simulink model "pitchPIDsimulation"  (R2025b)
settings: Solver=VariableStepAuto  StartTime=0.0  StopTime=15  RelTol=1e-3
undefined symbols (not defined in the file): CG, LongInertia, Mass, RotateInertia, Time
libraries: simulink x2, slpidlib x1
settings Model: Creator=Alienware R7  LastModifiedBy=Alienware R7

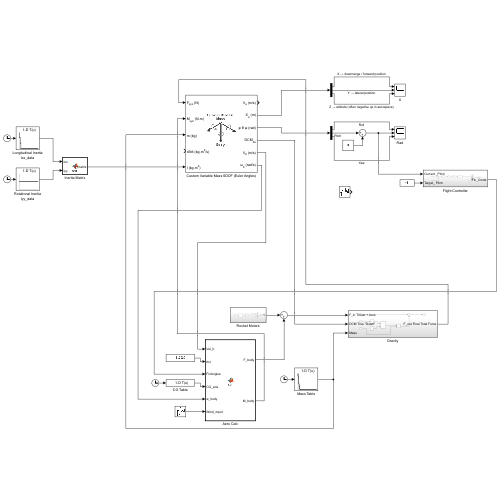
[thumbnail: Simulink's stored preview of the top-level diagram]
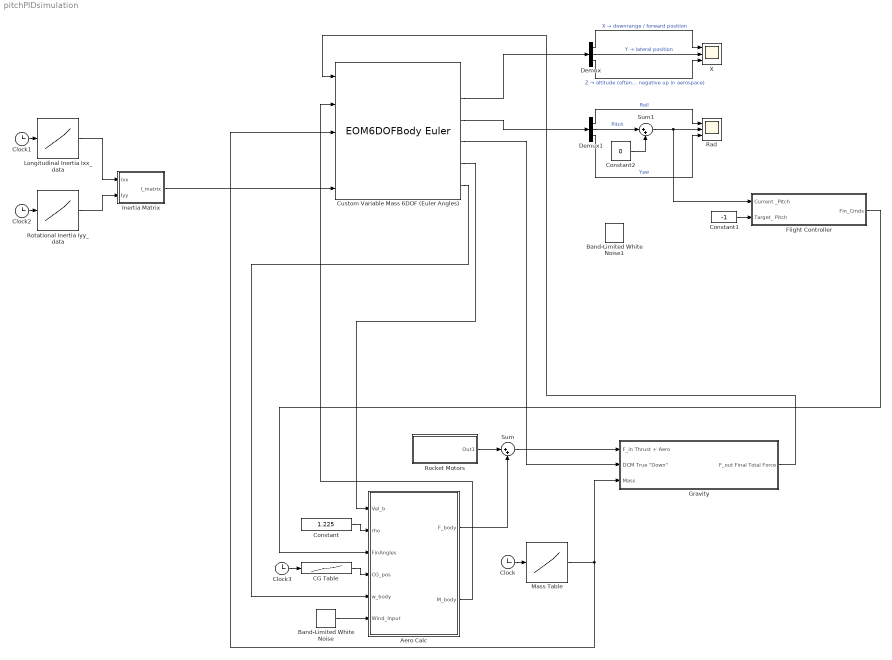
== system pitchPIDsimulation ==
  Aero Calc : MATLAB Function  TreatAsAtomicUnit=on
  Band-Limited White Noise : simulink/Sources/Band-Limited White Noise  Cov=0.1  Ts=0.05  seed=[23341]
  Band-Limited White Noise1 : simulink/Sources/Band-Limited White Noise  Cov=0.00005  Ts=0.01  seed=[23341]
  CG Table : Lookup_n-D  NumberOfTableDimensions=1  BreakpointsForDimension1=Time  Table=CG  InternalRulePriority=Speed  RndMeth=Simplest
  Clock{,1..3} (4 alike) : Clock
  Constant : Constant  Value=1.225
  Constant1 : Constant  Value=-1
  Constant2 : Constant  Value=0
  Custom Variable Mass 6DOF (Euler Angles) : EOM6DOFBodyEuler  mtype=Custom Variable  eul_0=[0 -0.75 0]
  Demux : Demux  Outputs=3
  Demux1 : Demux  Outputs=3
  Flight Controller : Subsystem
  Gravity : Subsystem
  Inertia Matrix : MATLAB Function  TreatAsAtomicUnit=on
  Longitudinal Inertia Ixx_data : Lookup_n-D  NumberOfTableDimensions=1  BreakpointsForDimension1=Time  Table=LongInertia  InternalRulePriority=Speed  RndMeth=Simplest
  Mass Table : Lookup_n-D  NumberOfTableDimensions=1  BreakpointsForDimension1=Time  Table=Mass  InternalRulePriority=Speed  RndMeth=Simplest
  Rad : Scope  NumInputPorts=3
      settings: ActiveDisplayYMinimum=-4.2416234281140159  ActiveDisplayYMaximum=2.850977580357458
  Rocket Motors : Subsystem
  Rotational Inertia Iyy_data : Lookup_n-D  NumberOfTableDimensions=1  BreakpointsForDimension1=Time  Table=RotateInertia  InternalRulePriority=Speed  RndMeth=Simplest
  Sum : Sum  Inputs=|++
  Sum1 : Sum  Inputs=|++
  X : Scope  NumInputPorts=3
      settings: ActiveDisplayYMinimum=-21.697738023426126  ActiveDisplayYMaximum=401.42440236350615
  wires:
  Rocket Motors/1(Out1) -> Sum/1
  Longitudinal Inertia Ixx_data/1 -> Inertia Matrix/1(Ixx)
  Rotational Inertia Iyy_data/1 -> Inertia Matrix/2(Iyy)
  Custom Variable Mass 6DOF (Euler Angles)/5 -> Aero Calc/1(Vel_b)
  CG Table/1 -> Aero Calc/4(CG_pos)
  Constant/1 -> Aero Calc/2(rho)
  Aero Calc/1(F_body) -> Sum/2
  Sum/1 -> Gravity/1(F_in Thrust + Aero)
  Custom Variable Mass 6DOF (Euler Angles)/4 -> Gravity/2("DCM True \"Down\"")
  Mass Table/1 -> Custom Variable Mass 6DOF (Euler Angles)/3, Gravity/3(Mass)
  Gravity/1(F_out Final Total Force) -> Custom Variable Mass 6DOF (Euler Angles)/1
  Clock/1 -> Mass Table/1
  Clock1/1 -> Longitudinal Inertia Ixx_data/1
  Clock2/1 -> Rotational Inertia Iyy_data/1
  Clock3/1 -> CG Table/1
  Inertia Matrix/1(I_matrix) -> Custom Variable Mass 6DOF (Euler Angles)/5
  Demux1/1 -> Rad/1  "Roll"
  Demux/2 -> X/2  "Y → lateral position"
  Demux1/3 -> Rad/3  "Yaw"
  Demux/3 -> X/3  "Z → altitude (often negative up in aerospace)"
  Demux/1 -> X/1  "X → downrange / forward position"
  Flight Controller/1(Fin_Cmds) -> Aero Calc/3(FinAngles)
  Aero Calc/2(M_body) -> Custom Variable Mass 6DOF (Euler Angles)/2
  Custom Variable Mass 6DOF (Euler Angles)/6 -> Aero Calc/5(w_body)
  Custom Variable Mass 6DOF (Euler Angles)/2 -> Demux/1
  Custom Variable Mass 6DOF (Euler Angles)/3 -> Demux1/1
  Demux1/2 -> Sum1/1  "Pitch"
  Sum1/1 -> Flight Controller/1(Current _Pitch), Rad/2
  Band-Limited White Noise/1 -> Aero Calc/6(Wind_Input)
  Constant1/1 -> Flight Controller/2(Target_ Pitch)
  Constant2/1 -> Sum1/2

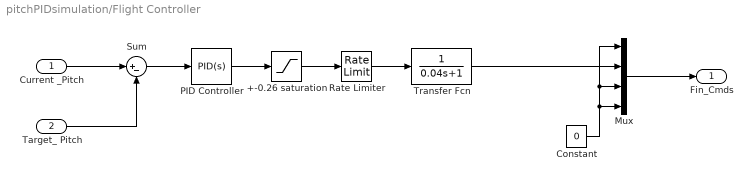
== system pitchPIDsimulation/Flight Controller ==
  Current _Pitch : Inport
  Target_ Pitch : Inport  Port=2
  +-0.26 saturation : Saturate  UpperLimit=0.26  LowerLimit=-0.26
  Constant : Constant  Value=0
  Mux : Mux
  PID Controller : slpidlib/PID Controller  Controller=PID  Form=Parallel  TimeDomain=Continuous-time  UseExternalTs=off  SampleTime=-1  IntegratorMethod=Forward Euler  FilterMethod=Forward Euler  ControllerParametersSource=internal  P=0.4  I=0  UseKiTs=off  D=0  UseExternalDerivativeSource=off  N=100  UseFilter=on  TunerSelectOption=Transfer Function Based (PID Tuner App)  InitialConditionSource=internal  InitialConditionForIntegrator=0  InitialConditionForFilter=0  DifferentiatorICPrevScaledInput=0  ExternalReset=none  TrackingMode=off  Kt=1  LimitOutput=off  SatLimitsSource=internal  UpperSaturationLimit=inf  LowerSaturationLimit=-inf  LinearizeAsGain=on  AntiWindupMode=none  Kb=1  LimitIntegrator=off  UpperIntegratorSaturationLimit=inf  LowerIntegratorSaturationLimit=-inf  POutMin=[]  POutMax=[]  IOutMin=[]  IOutMax=[]  DOutMin=[]  DOutMax=[]  NOutMin=[]  NOutMax=[]  SumOutMin=[]  SumOutMax=[]  SaturationOutMin=[]  SaturationOutMax=[]  PParamMin=[]  PParamMax=[]  IParamMin=[]  IParamMax=[]  DParamMin=[]  DParamMax=[]  NParamMin=[]  NParamMax=[]  KbParamMin=[]  KbParamMax=[]  KtParamMin=[]  KtParamMax=[]  KbOutMin=[]  KbOutMax=[]  KtOutMin=[]  KtOutMax=[]  IntegratorOutMin=[]  IntegratorOutMax=[]  FilterOutMin=[]  FilterOutMax=[]  SumI1OutMin=[]  SumI1OutMax=[]  SumI2OutMin=[]  SumI2OutMax=[]  SumI3OutMin=[]  SumI3OutMax=[]  SumI4OutMin=[]  SumI4OutMax=[]  SumDOutMin=[]  SumDOutMax=[]  DifferentiatorOutMin=[]  DifferentiatorOutMax=[]  FilterDiffOutCoefMin=[]  FilterDiffOutCoefMax=[]  ReciprocalOutMin=[]  ReciprocalOutMax=[]  SumDenOutMin=[]  SumDenOutMax=[]  SumNumOutMin=[]  SumNumOutMax=[]  DivideOutMin=[]  DivideOutMax=[]  UdiffTsProdOutMin=[]  UdiffTsProdOutMax=[]  NTsProdOutMin=[]  NTsProdOutMax=[]  UintegralTsProdOutMin=[]  UintegralTsProdOutMax=[]  UngainTsProdOutMin=[]  UngainTsProdOutMax=[]  ClampingZeroOutDataTypeStr=Inherit: Inherit via back propagation  ClampingZeroOutMin=[]  ClampingZeroOutMax=[]  FilterDenConstantOutDataTypeStr=Inherit: Inherit via back propagation  FilterDenConstantOutMin=[]  FilterDenConstantOutMax=[]  PCopyOutDataTypeStr=Inherit: Inherit via back propagation  PCopyOutMin=[]  PCopyOutMax=[]  NCopyOutDataTypeStr=Inherit: Inherit via back propagation  NCopyOutMin=[]  NCopyOutMax=[]  IntegratorContinuousStateAttributes=''  IntegratorStateMustResolveToSignalObject=off  IntegratorRTWStateStorageClass=Auto  FilterContinuousStateAttributes=''  FilterStateMustResolveToSignalObject=off  FilterRTWStateStorageClass=Auto  ParallelPVariant=InternalParameters  IdealPVariant=Disabled  IVariant=InternalParameters  DVariant=InternalParameters  IntegratorVariant=Continuous  SatVariant=Disabled  AWVariant=Passthrough  PCopyVariant=Disabled  TRVariant=Disabled  FdbkBlocksVariant=Forward  IdealPFdbkVariant=Disabled  SatFdbkVariant=Disabled  DerivativeFilterVariant=ContFilter  NVariant=InternalParameters  NCopyVariant=Disabled  FilterICVariant=InternalICsFilter  IntegratorICVariant=InternalICs  ExternalResetVariant=Disabled  TRSumVariant=Passthrough  SumFdbkVariant=Disabled  SumVariant=Sum_PID  TsampFilterVariant=InternalTs  TsampNgainVariant=Passthrough  TsampIntegralVariant=Disabled_SignalSpec  ExternalSaturationOutDataTypeStr=Inherit: Same as second input  DerivativeSourceVariant=ErrorSignal  PreIntVariant=InternalPreInt
  Rate Limiter : RateLimiter  RisingSlewLimit=8.05  FallingSlewLimit=-8.05  SampleTimeMode=inherited
  Sum : Sum  Inputs=|+-
  Transfer Fcn : TransferFcn  Denominator=[0.04 1]
  Fin_Cmds : Outport
  wires:
  Target_ Pitch/1 -> Sum/2
  Current _Pitch/1 -> Sum/1
  Sum/1 -> PID Controller/1
  PID Controller/1 -> +-0.26 saturation/1
  +-0.26 saturation/1 -> Rate Limiter/1
  Constant/1 -> Mux/3, Mux/1, Mux/4
  Mux/1 -> Fin_Cmds/1
  Rate Limiter/1 -> Transfer Fcn/1
  Transfer Fcn/1 -> Mux/2

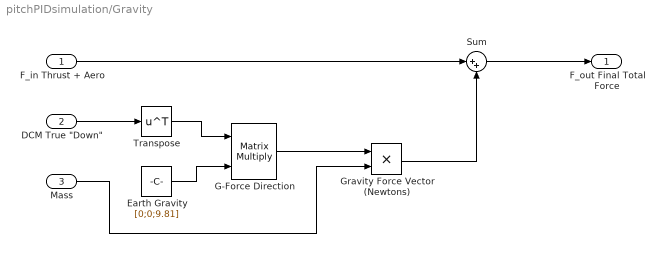
== system pitchPIDsimulation/Gravity ==
  F_in Thrust + Aero : Inport
  "DCM True \"Down\"" : Inport  Port=2
  Mass : Inport  Port=3
  Earth Gravity : Constant  Value=[0;0;9.81]
  G-Force Direction : Product  Multiplication=Matrix(*)
  Gravity Force Vector (Newtons) : Product
  Sum : Sum  Inputs=|++
  Transpose : Math  Operator=transpose
  F_out Final Total Force : Outport
  wires:
  "DCM True \"Down\""/1 -> Transpose/1
  Transpose/1 -> G-Force Direction/1
  Earth Gravity/1 -> G-Force Direction/2
  G-Force Direction/1 -> Gravity Force Vector (Newtons)/1
  Mass/1 -> Gravity Force Vector (Newtons)/2
  F_in Thrust + Aero/1 -> Sum/1
  Gravity Force Vector (Newtons)/1 -> Sum/2
  Sum/1 -> F_out Final Total Force/1

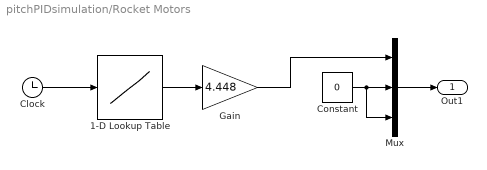
== system pitchPIDsimulation/Rocket Motors ==
  1-D Lookup Table : Lookup_n-D  NumberOfTableDimensions=1  BreakpointsForDimension1=[0;0.125;0.25;0.375;0.5;0.625;0.75;0.875;1;1.125;1.25;100]  Table=[0;31;36;41;41;46;55;60;58;50;0;0]  InternalRulePriority=Speed  RndMeth=Simplest
  Clock : Clock
  Constant : Constant  Value=0
  Gain : Gain  Gain=4.448
  Mux : Mux  Inputs=3
  Out1 : Outport
  wires:
  Clock/1 -> 1-D Lookup Table/1
  1-D Lookup Table/1 -> Gain/1
  Constant/1 -> Mux/2, Mux/3
  Gain/1 -> Mux/1
  Mux/1 -> Out1/1

== matlab function pitchPIDsimulation/Aero Calc ==
  data: Vel_b input; F_body output; rho input; FinAngles input; CG_pos input; M_body output; w_body input; Wind_Input input
function [F_body, M_body] = fcn(Vel_b, rho, FinAngles, CG_pos, w_body, Wind_Input)
    % --- 1. SETUP & WIND PHYSICS ---
    % ---------------------------------------------------------
    u = Vel_b(1); % Forward Velocity (Body X)
    w = Vel_b(3); % Down/Side Velocity (Body Z)
    q_rate = w_body(2); % Pitch Rate
    
    % [NEW] APPLY WIND DISTURBANCE
    % Wind_Input is lateral wind speed (m/s).
    % It adds to the "Side Velocity" the rocket feels.
    % If rocket is falling (w large) or wind hits (Wind_Input), both increase alpha.
    w_air = w + Wind_Input; 
    
    % CALCULATE TOTAL AIRSPEED (Magnitude)
    % We use w_air (relative to air), not w (relative to ground)
    V = sqrt(u^2 + w_air^2);
    
    % Prevent divide by zero / singularities at low speed
    if V < 0.1
        V = 0.1; 
    end
    
    
    % --- 2. ROCKET GEOMETRY ---
    % ---------------------------------------------------------
    L_rocket = 0.683;    
    D_rocket = 0.0762;   
    
    % Areas
    A_ref = pi * (D_rocket/2)^2;  % Front Cross-section (~0.00456 m^2)
    A_side = L_rocket * D_rocket; % Side Profile (~0.052 m^2)
    
    % YOUR FINS (Converted to m^2)
    % Rear: 12.5 in^2, Canard: 6.75 in^2
    % Total Pitch Area = 2 * (Rear + Canard)
    % Multiplier is 2 because only top/bottom fins act in pitch plane
    S_fins = 2 * (12.5 + 6.75) * 0.00064516; % ~0.0248 m^2
    
    X_cp = 0.421; % CP Location
    
    
    % --- 3. AERODYNAMICS ---
    % ---------------------------------------------------------
    q_dynamic = 0.5 * rho * V^2;
    
    % A. ANGLE OF ATTACK (ALPHA)
    % Calculated using Airspeed (w_air), so wind changes alpha!
    if V < 0.5
        alpha = 0;
    else
        alpha = atan2(w_air, u);
    end
    
    
    % B. DRAG (Directional Blend)
    % Drag always opposes the velocity vector.
    % As alpha increases (tumbling), Drag area blends from Front to Side.
    
    sin_alpha = abs(sin(alpha));
    
    % Blend Area: 0 deg = A_ref, 90 deg = A_side
    Current_Area = A_ref * (1 - sin_alpha) + A_side * sin_alpha;
    
    % Blend Cd: 0 deg = Nose Drag, 90 deg = Side Drag
    % Note: 2.2 is very high for nose drag (usually 0.5-0.75). 
    % If altitude is too low, lower this value.
    Current_Cd   = 2.2   * (1 - sin_alpha) + 1.2    * sin_alpha;
    
    Drag_Mag = q_dynamic * Current_Area * Current_Cd;
    
    % Drag Vector components (Opposite to Air Velocity)
    % We project the drag force back onto the body axes
    F_x_drag = -Drag_Mag * (u/V);
    F_z_drag = -Drag_Mag * (w_air/V);
    
    
    % C. LIFT (With Hard Stall)
    Total_Angle = alpha + FinAngles(2);
    
    % STALL LOGIC:
    % Real rockets stall sharply. If alpha > 15 deg (0.26 rad), 
    % the flow separates and Lift -> 0.
    % This prevents the "Glider" bug where tumbling rockets generate lift.
    
    if abs(Total_Angle) > 0.26 
        % STALLED / TUMBLING
        Cl = 0; 
    else
        % LINEAR LIFT (Flying)
        Cl_slope = 3.5;
        Cl = Cl_slope * Total_Angle;
    end
    
    % Lift Magnitude
    Lift_Mag = q_dynamic * S_fins * Cl;
    
    % Lift acts perpendicular to Velocity (roughly -Z in body frame)
    F_z_lift = -Lift_Mag;
    
    
    % --- 4. MOMENTS ---
    % ---------------------------------------------------------
    
    % Static Stability (The Spring)
    % Lever arm = Distance between CG and CP
    lever_arm = CG_pos(1) - X_cp; 
    M_pitch_static = Lift_Mag * lever_arm;
    
    % Damping (The Shock Absorber)
    % Rotational friction that stops infinite oscillation
    Damp_Factor = 0.5 * rho * V * S_fins * (L_rocket/2)^2;
    M_pitch_damp = -Damp_Factor * q_rate; 
    
    
    % --- 5. OUTPUTS ---
    % ---------------------------------------------------------
    F_body = [(F_x_drag); 0; (F_z_drag + F_z_lift)];
    M_body = [0; (M_pitch_static + M_pitch_damp); 0];
    
end

== matlab function pitchPIDsimulation/Inertia Matrix ==
  data: Ixx input; I_matrix output; Iyy input
function I_matrix = fcn(Ixx, Iyy)
    % Create a 3x3 Inertia Tensor
    % Rockets are symmetric, so we put Zeros in the corners.
    % Ixx is Roll Inertia. Iyy is Pitch/Yaw Inertia.
    
    I_matrix = [Ixx,  0,    0; 
                 0,  Iyy,   0; 
                 0,   0,   Iyy];
end
